simulink model "matsuoka_oscillator"  (Simulink 10.3)
settings: Solver=FixedStepAuto  StartTime=0.0  StopTime=10  FixedStep=0.02  MaxStep=1e-2  RelTol=1e-3  EnableMultiTasking=on
InitFcn:
  | init_param
StopFcn:
  | figure;
  | plot(tout, y1_out, 'b');
  | hold;
  | plot(tout, y2_out, 'r');
values from neighbouring files (symbols this model uses):
  b1 = 1.5    [init_param.m]    (also in threeNeuron_init_param.m)
  b2 = 1.5    [init_param.m]    (also in threeNeuron_init_param.m)
  q1 = 1    [init_param.m]    (also in tesArmTaga.m; threeNeuron_init_param.m)
  q2 = 1    [init_param.m]    (also in tesArmTaga.m; threeNeuron_init_param.m)
  Ta1 = 0.5    [init_param.m]    (also in tesArmTaga.m)
  Ta2 = 0.5    [init_param.m]    (also in tesArmTaga.m)
  Tr1 = 0.025    [init_param.m]    (also in tesArmTaga.m = 0.03125)
  Tr2 = 0.025    [init_param.m]    (also in tesArmTaga.m = 0.03125)
  w12 = 1.5    [init_param.m]    (also in tesArmTaga.m = 2; threeNeuron_init_param.m)
  w21 = 1.5    [init_param.m]    (also in tesArmTaga.m = 2; threeNeuron_init_param.m)
settings Model: Creator=manuruna  LastModifiedBy=HuijiangWang
settings DataIOCC: LimitDataPoints=on
settings DebuggingCC: SolverPrmCheckMsg=warning

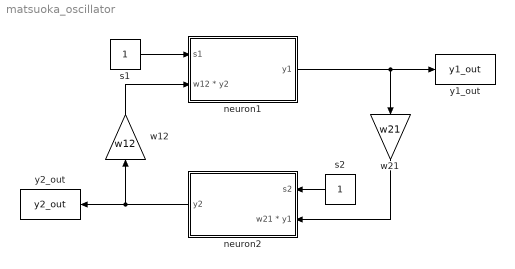
== system matsuoka_oscillator ==
  neuron1 : Subsystem
  neuron2 : Subsystem
  s1 : Constant
  s2 : Constant
  w12 : Gain  Gain=w12
  w21 : Gain  Gain=w21
  y1_out : ToWorkspace  VariableName=y1_out  SampleTime=-1
  y2_out : ToWorkspace  VariableName=y2_out  SampleTime=-1
  wires:
  w12/1 -> neuron1/2(w12 * y2)
  w21/1 -> neuron2/2(w21 * y1)
  neuron1/1(y1) -> w21/1, y1_out/1
  neuron2/1(y2) -> w12/1, y2_out/1
  s1/1 -> neuron1/1(s1)
  s2/1 -> neuron2/1(s2)

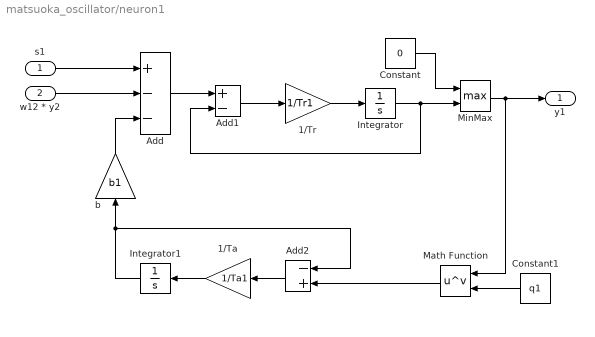
== system matsuoka_oscillator/neuron1 ==
  s1 : Inport
  w12 * y2 : Inport  Port=2
  1/Ta : Gain  Gain=1/Ta1
  1/Tr : Gain  Gain=1/Tr1
  Add : Sum  Inputs=+--
  Add1 : Sum  Inputs=+-
  Add2 : Sum  Inputs=-+
  Constant : Constant  Value=0
  Constant1 : Constant  Value=q1
  Integrator : Integrator
  Integrator1 : Integrator
  Math Function : Math  Operator=pow  SignedPower=on  OutputSignalType=real  SaturateOnIntegerOverflow=on
  MinMax : MinMax  Function=max  Inputs=2
  b : Gain  Gain=b1
  y1 : Outport
  wires:
  s1/1 -> Add/1
  w12 * y2/1 -> Add/2
  Add/1 -> Add1/1
  Add1/1 -> 1/Tr/1
  1/Tr/1 -> Integrator/1
  Integrator/1 -> MinMax/2, Add1/2
  Constant/1 -> MinMax/1
  MinMax/1 -> y1/1, Math Function/1
  b/1 -> Add/3
  Add2/1 -> 1/Ta/1
  1/Ta/1 -> Integrator1/1
  Integrator1/1 -> b/1, Add2/1
  Math Function/1 -> Add2/2
  Constant1/1 -> Math Function/2

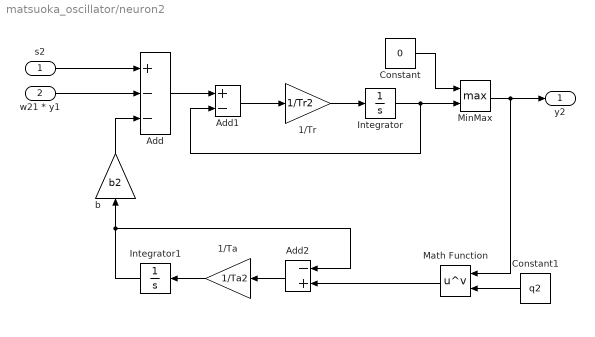
== system matsuoka_oscillator/neuron2 ==
  s2 : Inport
  w21 * y1 : Inport  Port=2
  1/Ta : Gain  Gain=1/Ta2
  1/Tr : Gain  Gain=1/Tr2
  Add : Sum  Inputs=+--
  Add1 : Sum  Inputs=+-
  Add2 : Sum  Inputs=-+
  Constant : Constant  Value=0
  Constant1 : Constant  Value=q2
  Integrator : Integrator
  Integrator1 : Integrator
  Math Function : Math  Operator=pow  SignedPower=on  OutputSignalType=real  SaturateOnIntegerOverflow=on
  MinMax : MinMax  Function=max  Inputs=2
  b : Gain  Gain=b2
  y2 : Outport
  wires:
  Integrator1/1 -> Add2/1, b/1
  1/Ta/1 -> Integrator1/1
  Add2/1 -> 1/Ta/1
  b/1 -> Add/3
  MinMax/1 -> y2/1, Math Function/1
  Constant/1 -> MinMax/1
  Integrator/1 -> Add1/2, MinMax/2
  1/Tr/1 -> Integrator/1
  Add1/1 -> 1/Tr/1
  Add/1 -> Add1/1
  w21 * y1/1 -> Add/2
  s2/1 -> Add/1
  Math Function/1 -> Add2/2
  Constant1/1 -> Math Function/2
